simulink model "upravljanjeBrzinom2012a"  (R2012a)
settings: Solver=ode3  SolverMode=SingleTasking  StartTime=0.0  StopTime=100  RelTol=1e-3
values from neighbouring files (symbols this model uses):
  b = 0.7    [konstanteBrzina.m]    (also in konstantePozicija.m = 1)
  K1 = 0.3    [konstanteBrzina.m]
  K2 = 0.1    [konstanteBrzina.m]
  Km = 180    [konstanteBrzina.m]
  N = 3    [konstanteBrzina.m]    (also in konstantePozicija.m = 8)
  T = 0.01    [konstanteBrzina.m]    (also in konstantePozicija.m)
  Td2 = 0.06    [konstanteBrzina.m]
  Ti1 = 1.3    [konstanteBrzina.m]
  Ti2 = 0.8    [konstanteBrzina.m]
  Tm = 1.3    [konstanteBrzina.m]
settings Model: CovMetricSettings=dwe  CovHtmlReporting=off  covSaveCumulativeToWorkspaceVar=off  CovSaveSingleToWorkspaceVar=off  CovExternalEMLEnable=on  Creator=Anja  LastModifiedBy=Anja
settings DataIOCC: SaveFormat=StructureWithTime  ReturnWorkspaceOutputs=off
settings OptimizationCC: LifeSpan=inf  SimCompilerOptimization=Off
settings DebuggingCC: FcnCallInpInsideContextMsg=Enable All
settings HardwareCC: ProdWordSize=32  ProdHWDeviceType=Specified
settings SFSimCC: SimUseLocalCustomCode=off
settings RTWCC: RTWUseLocalCustomCode=off  RTWCompilerOptimization=Off
settings GRTTargetCC: CodeReplacementLibrary=C99 (ISO)  CPPClassGenCompliant=off

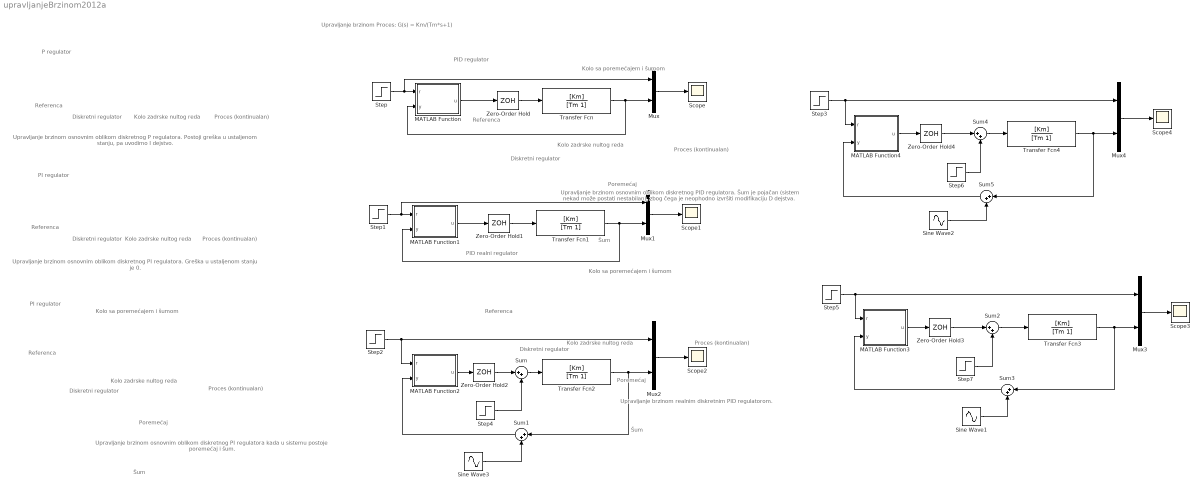
== system upravljanjeBrzinom2012a ==
  note: Upravljanje brzinom
      | Proces: G(s) = Km/(Tm*s+1)
  note: P regulator
  note: PI regulator
  note: PI regulator
  note: Kolo sa poremećajem i šumom
  note: Kolo sa poremećajem i šumom
  note: PID realni regulator
  note: Kolo sa poremećajem i šumom
  note: PID regulator
  note: Upravljanje brzinom osnovnim oblikom diskretnog P regulatora. Postoji greška u ustaljenom stanju, pa uvodimo I dejstvo.
  note: Upravljanje brzinom osnovnim oblikom diskretnog PI regulatora. Greška u ustaljenom stanju je 0.
  note: Upravljanje brzinom osnovnim oblikom diskretnog PI regulatora kada u sistemu postoje poremećaj i šum.
  note: Upravljanje brzinom osnovnim oblikom diskretnog PID regulatora. Šum je pojačan (sistem nekad može postati nestabilan), zbog čega je neophodno izvršiti modifikaciju D dejstva.
  note: Upravljanje brzinom realnim diskretnim PID regulatorom.
  note: Proces (kontinualan)
  note: Diskretni regulator
  note: Referenca
  note: Kolo zadrske nultog reda
  note: Referenca
  note: Referenca
  note: Referenca
  note: Referenca
  note: Diskretni regulator
  note: Diskretni regulator
  note: Diskretni regulator
  note: Diskretni regulator
  note: Proces (kontinualan)
  note: Proces (kontinualan)
  note: Proces (kontinualan)
  note: Proces (kontinualan)
  note: Kolo zadrske nultog reda
  note: Kolo zadrske nultog reda
  note: Kolo zadrske nultog reda
  note: Kolo zadrske nultog reda
  note: Poremećaj
  note: Poremećaj
  note: Poremećaj
  note: Šum
  note: Šum
  note: Šum
  MATLAB Function : MATLAB Function  TreatAsAtomicUnit=on
      settings: PermitHierarchicalResolution=ParametersOnly
  MATLAB Function1 : MATLAB Function  TreatAsAtomicUnit=on
      settings: PermitHierarchicalResolution=ParametersOnly
  MATLAB Function2 : MATLAB Function  TreatAsAtomicUnit=on
      settings: PermitHierarchicalResolution=ParametersOnly
  MATLAB Function3 : MATLAB Function  TreatAsAtomicUnit=on
      settings: PermitHierarchicalResolution=ParametersOnly
  MATLAB Function4 : MATLAB Function  TreatAsAtomicUnit=on
      settings: PermitHierarchicalResolution=ParametersOnly
  Mux{,1..4} (5 alike) : Mux  Inputs=2
  Scope{,1..4} (5 alike) : Scope
      Scope settings: TimeRange=auto  MaxDataPoints=5000  SaveToWorkspace=off  SaveName=ScopeData  YMin=-17.5  YMax=157.5  SampleTime=-1
      Scope1 settings: TimeRange=auto  MaxDataPoints=5000  SaveToWorkspace=off  YMin=-17.93252  YMax=161.3927  SampleTime=-1
      Scope2 settings: TimeRange=auto  MaxDataPoints=5000  SaveToWorkspace=off  YMin=-1.66183  YMax=14.69042  SampleTime=-1
      Scope3 settings: TimeRange=auto  MaxDataPoints=5000  SaveToWorkspace=off  YMin=9.96211  YMax=10.03743  SampleTime=-1
      Scope4 settings: TimeRange=auto  MaxDataPoints=5000  SaveToWorkspace=off  YMin=9.94633  YMax=10.05098  SampleTime=-1
  Sine Wave1 : Sin  Amplitude=0.1  Frequency=50000  SampleTime=0
  Sine Wave2 : Sin  Amplitude=0.1  Frequency=50000  SampleTime=0
  Sine Wave3 : Sin  Amplitude=0.1  Frequency=50000  SampleTime=0
  Step : Step  After=140  SampleTime=0
  Step1 : Step  After=140  SampleTime=0
  Step2 : Step  After=10  SampleTime=0
  Step3 : Step  After=10  SampleTime=0
  Step4 : Step  Time=5  SampleTime=0
  Step5 : Step  After=10  SampleTime=0
  Step6 : Step  Time=5  SampleTime=0
  Step7 : Step  Time=5  SampleTime=0
  Sum{,1..5} (6 alike) : Sum  Inputs=|++
  Transfer Fcn{,1..4} (5 alike) : TransferFcn  Numerator=[Km]  Denominator=[Tm 1]
  Zero-Order Hold{,1..4} (5 alike) : ZeroOrderHold  SampleTime=T
  wires:
  MATLAB Function/1(u) -> Zero-Order Hold/1
  Step/1 -> Mux/1, MATLAB Function/1(r)
  Mux/1 -> Scope/1
  Transfer Fcn/1 -> Mux/2, MATLAB Function/2(y)
  Step1/1 -> Mux1/1, MATLAB Function1/1(r)
  MATLAB Function1/1(u) -> Zero-Order Hold1/1
  Transfer Fcn1/1 -> Mux1/2, MATLAB Function1/2(y)
  Mux1/1 -> Scope1/1
  Step2/1 -> MATLAB Function2/1(r), Mux2/1
  Mux2/1 -> Scope2/1
  MATLAB Function2/1(u) -> Zero-Order Hold2/1
  Sum/1 -> Transfer Fcn2/1
  Step4/1 -> Sum/2
  Sum1/1 -> MATLAB Function2/2(y)
  Transfer Fcn2/1 -> Mux2/2, Sum1/1
  Transfer Fcn3/1 -> Mux3/2, Sum3/1
  Step7/1 -> Sum2/2
  Sine Wave1/1 -> Sum3/2
  Step5/1 -> Mux3/1, MATLAB Function3/1(r)
  Sum2/1 -> Transfer Fcn3/1
  Sum3/1 -> MATLAB Function3/2(y)
  Mux3/1 -> Scope3/1
  Zero-Order Hold/1 -> Transfer Fcn/1
  Zero-Order Hold1/1 -> Transfer Fcn1/1
  Zero-Order Hold2/1 -> Sum/1
  Zero-Order Hold3/1 -> Sum2/1
  Zero-Order Hold4/1 -> Sum4/1
  Sum4/1 -> Transfer Fcn4/1
  Step3/1 -> MATLAB Function4/1(r), Mux4/1
  MATLAB Function4/1(u) -> Zero-Order Hold4/1
  Sum5/1 -> MATLAB Function4/2(y)
  Transfer Fcn4/1 -> Mux4/2, Sum5/1
  Mux4/1 -> Scope4/1
  Sine Wave2/1 -> Sum5/2
  Step6/1 -> Sum4/2
  MATLAB Function3/1(u) -> Zero-Order Hold3/1
  Sine Wave3/1 -> Sum1/2

== matlab function upravljanjeBrzinom2012a/MATLAB Function1 ==
  settings: updateMethod=DISCRETE
  data: u output; r input; y input; K1 parameter; T parameter; Ti1 parameter
function u = fcn(r, y, K1, T, Ti1)
% implementacija osnovnog oblika diskretnog PI regulatora
% Ulazni parametri su: r - referenca, y - izlaz iz sistema (procesa), K1 -
% proporcionalno pojacanje, T - perioda odabiranja, Ti1 - vremenska konstantna integraljenja.
% Izlazni parametar je upravljanje: u = P + I.
% I dejstvo je diskretizovano diferenciranjem unazad I(kT + T) = I(kT) + (K1*T/Ti1)*e(kT)
% I(kT) = I(kT-T) + K1*T*(r(kT-T) - y(kT-T))/Ti1
% Za cuvanje prethodnih vrednosti neke promenljive, izmedju poziva f-je,
% koristi se funkacije persistent. Pogledati help persistent

persistent Ip; % I(kT-T)
persistent yp; % y(kT-T)
persistent rp; % r(kT-T)

% Inicijalizacija perzistentnih promeniljivih Ip, yp i rp na nulu ukoliko su
% prazne (npr. na pocetku)
if (isempty(Ip))
    Ip=0;
end

if (isempty(yp))
    yp=0;
end

if (isempty(rp))
    rp=0;
end

P = K1 * (r - y); % deo upravljanja - P dejstvo
I = Ip + K1*T*(rp - yp)/Ti1; % I dejstvo
u = P + I; % ukupno upravljanje

% azuriranje promenljivih
Ip = I;
yp=y;
rp=r;

end

== matlab function upravljanjeBrzinom2012a/MATLAB Function ==
  data: u output; r input; y input; K parameter
function u = fcn(r, y, K)
% implementacija osnovnog oblika diskretnog P regulatora
% Ulazni parametri su: r - referenca, y - izlaz iz sistema (procesa), K -
% proporcionalno pojacanje.
% Izlazni parametar je upravljanje: u = P = Ke = K(r-y).

u = K * (r - y);

end

== matlab function upravljanjeBrzinom2012a/MATLAB Function2 ==
  settings: updateMethod=DISCRETE
  data: u output; r input; y input; K1 parameter; T parameter; Ti1 parameter
function u = fcn(r, y, K1, T, Ti1)
% implementacija osnovnog oblika diskretnog PI regulatora
% Ulazni parametri su: r - referenca, y - izlaz iz sistema (procesa), K1 -
% proporcionalno pojacanje, T - perioda odabiranja, Ti1 - vremenska konstantna integraljenja.
% Izlazni parametar je upravljanje: u = P + I.
% I dejstvo je diskretizovano diferenciranjem unazad I(kT + T) = I(kT) + (K1*T/Ti1)*e(kT)
% I(kT) = I(kT-T) + K1*T*(r(kT-T) - y(kT-T))/Ti1
% Za cuvanje prethodnih vrednosti neke promenljive, izmedju poziva f-je,
% koristi se funkacije persistent. Pogledati help persistent

persistent Ip; % I(kT-T)
persistent yp; % y(kT-T)
persistent rp; % r(kT-T)

% Inicijalizacija perzistentnih promeniljivih Ip, yp i rp na nulu ukoliko su
% prazne (npr. na pocetku)

if (isempty(Ip))
    Ip=0;
end

if (isempty(yp))
    yp=0;
end

if (isempty(rp))
    rp=0;
end

P = K1 * (r - y); % deo upravljanja - P dejstvo
I = Ip + K1*T*(rp - yp)/Ti1; % I dejstvo
u = P + I; % ukupno upravljanje

% azuriranje promenljivih
Ip = I;
yp=y;
rp=r;

end

== matlab function upravljanjeBrzinom2012a/MATLAB Function3 ==
  settings: updateMethod=DISCRETE
  data: u output; r input; y input; K2 parameter; T parameter; Ti2 parameter; b parameter; Td2 parameter; N parameter
function u = fcn(r, y, K2, T, Ti2, b, Td2, N)
% implementacija realnog diskretnog PID regulatora
% Ulazni parametri su: r - referenca, y - izlaz iz sistema (procesa), K2 -
% proporcionalno pojacanje, T - perioda odabiranja, Ti2 - vremenska
% konstantna integraljenja, Td2 - vremenska konstanta diferenciranja, 
% N - vremenska konstanta niskopropusnog filtra, b - tezinski faktor.
% Izlazni parametar je upravljanje: u = P + I + D.
% I dejstvo je diskretizovano diferenciranjem unazad I(kT + T) = I(kT) + (K1*T/Ti1)*e(kT)
% I(kT) = I(kT-T) + K1*T*(r(kT-T) - y(kT-T))/Ti1
% D dejstvo je tkdj. diskretizovano diferenciranjem unazad
% D(kT) = (Td2/(Td2 + N*T))*D(kT-T) - (K2 * Td2*N)/(Td2+N*T*(y(kT)-y(kT-T))
% Za cuvanje prethodnih vrednosti neke promenljive, izmedju poziva f-je,
% koristi se funkacije persistent. Pogledati help persistent

persistent Ip; % I(kT-T)
persistent yp; % y(kT-T)
persistent rp; % r(kT-T)
persistent Dp; % D(kT-T)

% Inicijalizacija perzistentnih promeniljivih Ip, yp i rp na nulu ukoliko su
% prazne (npr. na pocetku)

if (isempty(Ip))
    Ip=0;
end

if (isempty(Dp))
    Dp=0;
end

if (isempty(yp))
    yp=0;
end

if (isempty(rp))
    rp=0;
end

P = K2 * (b*r - y); % deo upravljanja - P dejstvo
I = Ip + K2*T*(rp - yp)/Ti2; % I dejstvo
c = Td2/(Td2 + N*T); % konstanta
d = (K2 * Td2*N)/(Td2+N*T); % kon
D = c*Dp - d*(y-yp); % D dejstvo
u = P + I + D;

% azuriranje promenljivih
Ip = I;
yp=y;
rp=r;
Dp = D;

end

== matlab function upravljanjeBrzinom2012a/MATLAB Function4 ==
  settings: updateMethod=DISCRETE
  data: u output; r input; y input; K2 parameter; T parameter; Ti2 parameter; Td2 parameter
function u = fcn(r, y, K2, T, Ti2, Td2)
% implementacija osnovnog oblika diskretnog PID regulatora
% Ulazni parametri su: r - referenca, y - izlaz iz sistema (procesa), K2 -
% proporcionalno pojacanje, T - perioda odabiranja, Ti2 - vremenska
% konstantna integraljenja, Td2 - vremenska konstanta diferenciranja.
% Izlazni parametar je upravljanje: u = P + I + D.
% I dejstvo je diskretizovano diferenciranjem unazad I(kT + T) = I(kT) + (K1*T/Ti1)*e(kT)
% I(kT) = I(kT-T) + K1*T*(r(kT-T) - y(kT-T))/Ti1
% D dejstvo je tkdj. diskretizovano diferenciranjem unazad
% D(kT) = K2*Td2*(y(kT) - y(kT-T))/T
% Za cuvanje prethodnih vrednosti neke promenljive, izmedju poziva f-je,
% koristi se funkacije persistent. Pogledati help persistent

persistent Ip; % I(kT-T)
persistent yp; % y(kT-T)
persistent rp; % r(kT-T)

% Inicijalizacija perzistentnih promeniljivih Ip, yp i rp na nulu ukoliko su
% prazne (npr. na pocetku)

if (isempty(Ip))
    Ip=0;
end

if (isempty(yp))
    yp=0;
end

if (isempty(rp))
    rp=0;
end

P = K2 * (r - y); % deo upravljanja - P dejstvo
I = Ip + K2*T*(rp - yp)/Ti2; % I dejstvo
D = K2*Td2*(y - yp)/T; % D dejstvo
u = P + I + D; % ukupno upravljanje

% azuriranje promenljivih
Ip = I;
yp=y;
rp=r;

end
